simulink model "Worked_Example_8_3"  (R2024b)
settings: Solver=VariableStepAuto  StartTime=0.0  StopTime=10  RelTol=1e-3
settings Model: Creator=GH-X-ST  LastModifiedBy=GH-X-ST

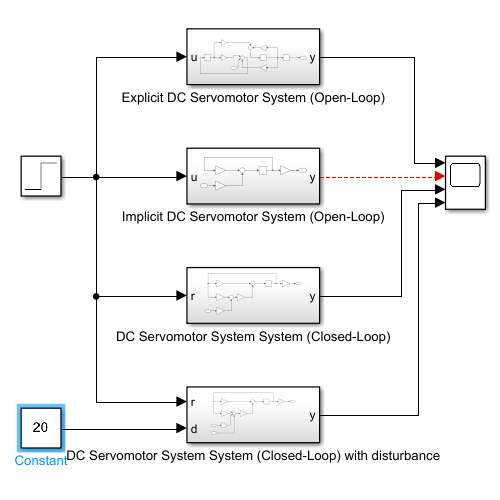
[thumbnail: Simulink's stored preview of the top-level diagram]
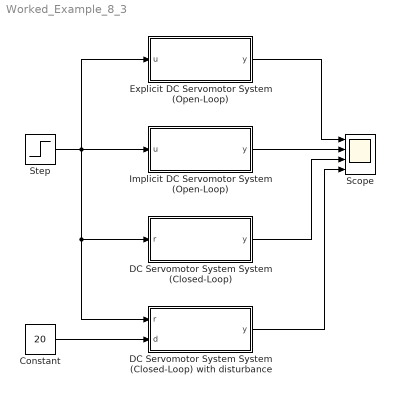
== system Worked_Example_8_3 ==
  Constant : Constant  Value=20
  DC Servomotor System System (Closed-Loop) : Subsystem
  DC Servomotor System System (Closed-Loop) with disturbance : Subsystem
  Explicit DC Servomotor System (Open-Loop) : Subsystem
  Implicit DC Servomotor System (Open-Loop) : Subsystem
  Scope : Scope  NumInputPorts=4
  Step : Step  SampleTime=0
  wires:
  Explicit DC Servomotor System (Open-Loop)/1(y) -> Scope/1
  Step/1 -> DC Servomotor System System (Closed-Loop) with disturbance/1(r), DC Servomotor System System (Closed-Loop)/1(r), Explicit DC Servomotor System (Open-Loop)/1(u), Implicit DC Servomotor System (Open-Loop)/1(u)
  DC Servomotor System System (Closed-Loop)/1(y) -> Scope/3
  Implicit DC Servomotor System (Open-Loop)/1(y) -> Scope/2
  DC Servomotor System System (Closed-Loop) with disturbance/1(y) -> Scope/4
  Constant/1 -> DC Servomotor System System (Closed-Loop) with disturbance/2(d)

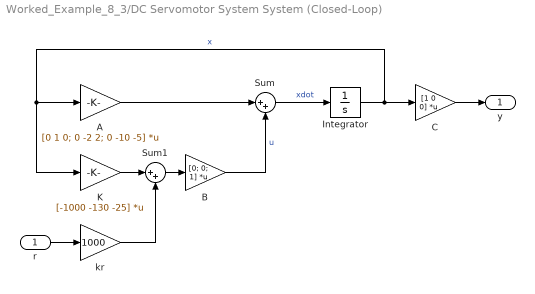
== system Worked_Example_8_3/DC Servomotor System System (Closed-Loop) ==
  r : Inport
  A : Gain  Gain=[0 1 0; 0 -2 2; 0 -10 -5]  Multiplication=Matrix(K*u)
  B : Gain  Gain=[0; 0; 1]  Multiplication=Matrix(K*u)
  C : Gain  Gain=[1 0 0]  Multiplication=Matrix(K*u)
  Integrator : Integrator
  K : Gain  Gain=[-1000 -130 -25]  Multiplication=Matrix(K*u)
  Sum : Sum  Inputs=|++
  Sum1 : Sum  Inputs=|++
  kr : Gain  Gain=1000
  y : Outport
  wires:
  C/1 -> y/1
  Integrator/1 -> C/1, K/1, A/1  "x"
  Sum/1 -> Integrator/1  "xdot"
  A/1 -> Sum/1
  r/1 -> kr/1
  K/1 -> Sum1/1
  Sum1/1 -> B/1
  kr/1 -> Sum1/2
  B/1 -> Sum/2  "u"

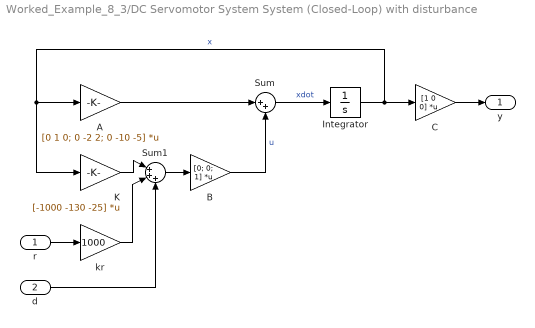
== system Worked_Example_8_3/DC Servomotor System System (Closed-Loop) with disturbance ==
  r : Inport
  d : Inport  Port=2
  A : Gain  Gain=[0 1 0; 0 -2 2; 0 -10 -5]  Multiplication=Matrix(K*u)
  B : Gain  Gain=[0; 0; 1]  Multiplication=Matrix(K*u)
  C : Gain  Gain=[1 0 0]  Multiplication=Matrix(K*u)
  Integrator : Integrator
  K : Gain  Gain=[-1000 -130 -25]  Multiplication=Matrix(K*u)
  Sum : Sum  Inputs=|++
  Sum1 : Sum  Inputs=|+++
  kr : Gain  Gain=1000
  y : Outport
  wires:
  C/1 -> y/1
  Integrator/1 -> C/1, K/1, A/1  "x"
  Sum/1 -> Integrator/1  "xdot"
  A/1 -> Sum/1
  r/1 -> kr/1
  K/1 -> Sum1/1
  Sum1/1 -> B/1
  kr/1 -> Sum1/2
  B/1 -> Sum/2  "u"
  d/1 -> Sum1/3

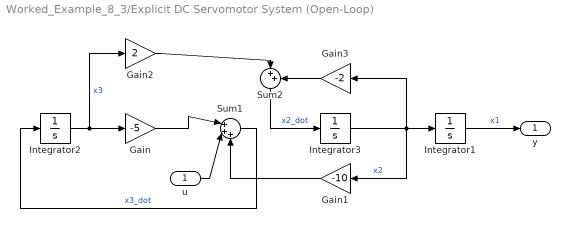
== system Worked_Example_8_3/Explicit DC Servomotor System (Open-Loop) ==
  u : Inport
  Gain : Gain  Gain=-5
  Gain1 : Gain  Gain=-10
  Gain2 : Gain  Gain=2
  Gain3 : Gain  Gain=-2
  Integrator1 : Integrator
  Integrator2 : Integrator
  Integrator3 : Integrator
  Sum1 : Sum  Inputs=|+++
  Sum2 : Sum  Inputs=|++
  y : Outport
  wires:
  Integrator3/1 -> Gain1/1, Gain3/1, Integrator1/1  "x2"
  Integrator1/1 -> y/1  "x1"
  u/1 -> Sum1/2
  Integrator2/1 -> Gain2/1, Gain/1  "x3"
  Sum1/1 -> Integrator2/1  "x3_dot"
  Gain/1 -> Sum1/1
  Gain1/1 -> Sum1/3
  Sum2/1 -> Integrator3/1  "x2_dot"
  Gain2/1 -> Sum2/1
  Gain3/1 -> Sum2/2

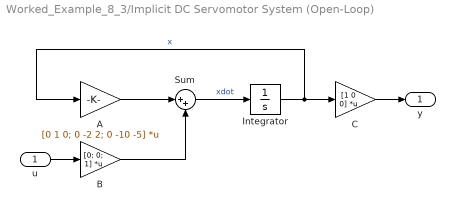
== system Worked_Example_8_3/Implicit DC Servomotor System (Open-Loop) ==
  u : Inport
  A : Gain  Gain=[0 1 0; 0 -2 2; 0 -10 -5]  Multiplication=Matrix(K*u)
  B : Gain  Gain=[0; 0; 1]  Multiplication=Matrix(K*u)
  C : Gain  Gain=[1 0 0]  Multiplication=Matrix(K*u)
  Integrator : Integrator
  Sum : Sum  Inputs=|++
  y : Outport
  wires:
  u/1 -> B/1
  A/1 -> Sum/1
  B/1 -> Sum/2
  Sum/1 -> Integrator/1  "xdot"
  Integrator/1 -> C/1, A/1  "x"
  C/1 -> y/1
